simulink model "Prob03"  (R2020a)
settings: Solver=ode45  StartTime=0.0  StopTime=120  RelTol=1e-3
InitFcn:
  | m = 1000;
  | b = 50;
  | u = 500;
settings Model: Creator=Shivam  LastModifiedBy=Shivam

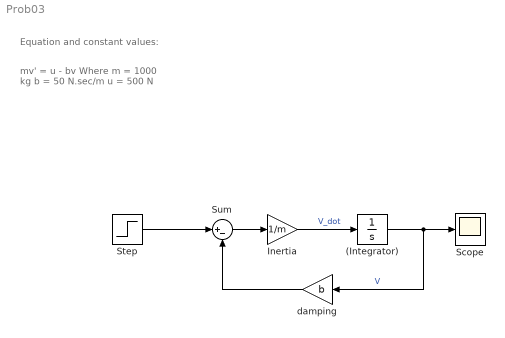
== system Prob03 ==
  note: mv' = u - bv
      |
      | Where
      | m = 1000 kg
      | b = 50 N.sec/m
      | u = 500 N
  note: Equation and constant values:
  (Integrator) : Integrator
  Inertia : Gain  Gain=1/m
  Scope : Scope
  Step : Step  Time=0  After=u  SampleTime=0
  Sum : Sum  Inputs=|+-
  damping : Gain  Gain=b
  wires:
  Inertia/1 -> (Integrator)/1  "V_dot"
  (Integrator)/1 -> Scope/1, damping/1  "V"
  Sum/1 -> Inertia/1
  damping/1 -> Sum/2
  Step/1 -> Sum/1
